simulink subsystem "Strecke"  (R2021b)
settings: Solver=VariableStepAuto  StartTime=0.0  StopTime=10.0  RelTol=1e-3
undefined symbols (not defined in the file or in its folder): SimParam
settings Model: Creator=tim  LastModifiedBy=tim

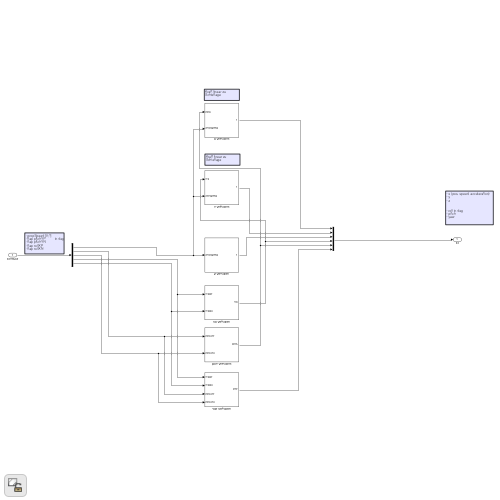
[thumbnail: Simulink's stored preview of the top-level diagram]
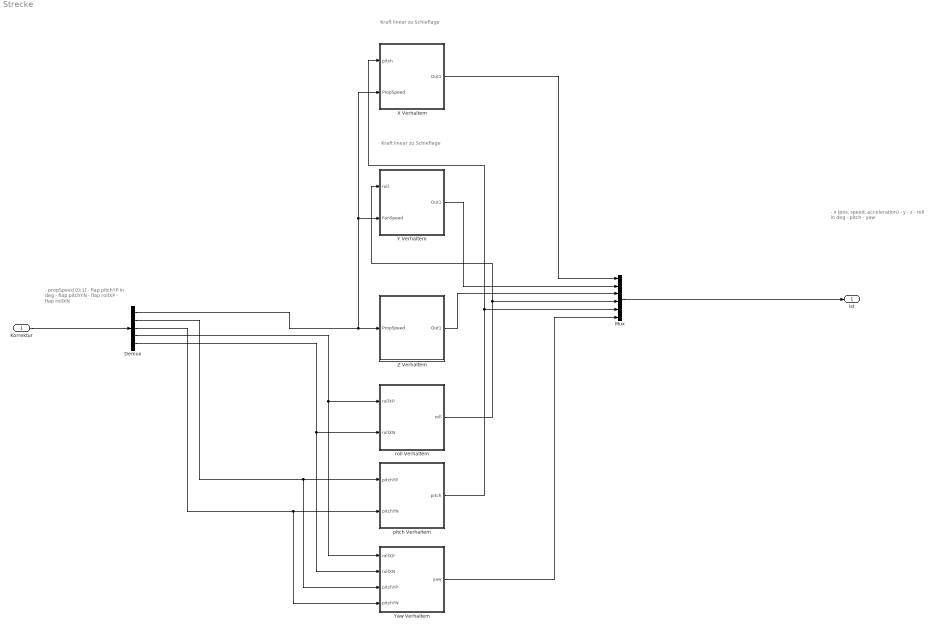
== system Strecke ==
  note: Kraft linear zu
      | Schieflage
  note: - propSpeed [0;1]
      | - flap pitchYP          in deg
      | - flap pitchYN
      | - flap rollXP
      | - flap rollXN
  note: - x (pos, speed, acceleration)
      | - y
      | - z
      |
      |
      | - roll in deg
      | - pitch
      | - yaw
  note: Kraft linear zu
      | Schieflage
  Korrektur : Inport
  Demux : Demux  Outputs=5
  Mux : Mux  Inputs=6
  X Verhaltem : Subsystem
  Y Verhaltem : Subsystem
  Yaw Verhaltem : Subsystem
  Z Verhaltem : Subsystem
  pitch Verhaltem : Subsystem
  roll Verhaltem : Subsystem
  ist : Outport
  wires:
  Demux/1 -> Z Verhaltem/1(PropSpeed), Y Verhaltem/2(FanSpeed), X Verhaltem/2(PropSpeed)
  Z Verhaltem/1(Out1) -> Mux/3
  Korrektur/1 -> Demux/1
  X Verhaltem/1(Out1) -> Mux/1
  Y Verhaltem/1(Out1) -> Mux/2
  Demux/2 -> pitch Verhaltem/1(pitchYP), Yaw Verhaltem/3(pitchYP)
  Demux/3 -> pitch Verhaltem/2(pitchYN), Yaw Verhaltem/4(pitchYN)
  Demux/4 -> roll Verhaltem/1(rollXP), Yaw Verhaltem/1(rollXP)
  Demux/5 -> roll Verhaltem/2(rollXN), Yaw Verhaltem/2(rollXN)
  roll Verhaltem/1(roll) -> Y Verhaltem/1(roll), Mux/4
  Yaw Verhaltem/1(yaw) -> Mux/6
  pitch Verhaltem/1(pitch) -> X Verhaltem/1(pitch), Mux/5
  Mux/1 -> ist/1

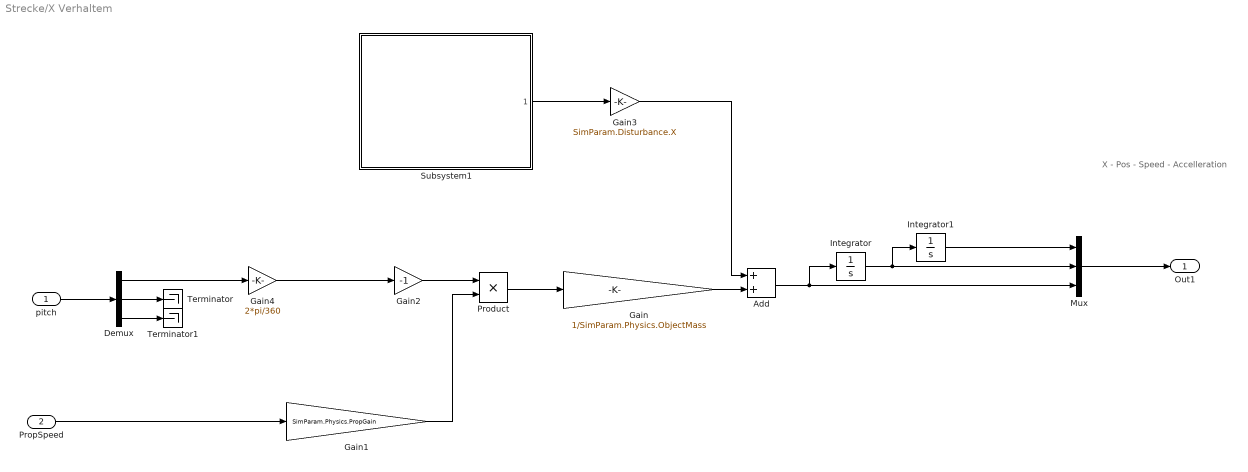
== system Strecke/X Verhaltem ==
  note: X
      | - Pos
      | - Speed
      | - Accelleration
  pitch : Inport
  PropSpeed : Inport  Port=2
  Add : Sum
  Demux : Demux  Outputs=3
  Gain : Gain  Gain=1/SimParam.Physics.ObjectMass
  Gain1 : Gain  Gain=SimParam.Physics.PropGain
  Gain2 : Gain  Gain=-1
  Gain3 : Gain  Gain=SimParam.Disturbance.X
  Gain4 : Gain  Gain=2*pi/360
  Integrator : Integrator
  Integrator1 : Integrator
  Mux : Mux  Inputs=3
  Product : Product
  Subsystem1 : Subsystem  ReferencedSubsystem=Disturbance
  Terminator : Terminator
  Terminator1 : Terminator
  Out1 : Outport
  wires:
  Gain2/1 -> Product/1
  Gain4/1 -> Gain2/1
  Gain1/1 -> Product/2
  PropSpeed/1 -> Gain1/1
  Gain3/1 -> Add/1
  Subsystem1/1 -> Gain3/1
  Gain/1 -> Add/2
  Demux/1 -> Gain4/1
  Demux/3 -> Terminator1/1
  Demux/2 -> Terminator/1
  Product/1 -> Gain/1
  Add/1 -> Mux/3, Integrator/1
  Integrator1/1 -> Mux/1
  Integrator/1 -> Mux/2, Integrator1/1
  pitch/1 -> Demux/1
  Mux/1 -> Out1/1

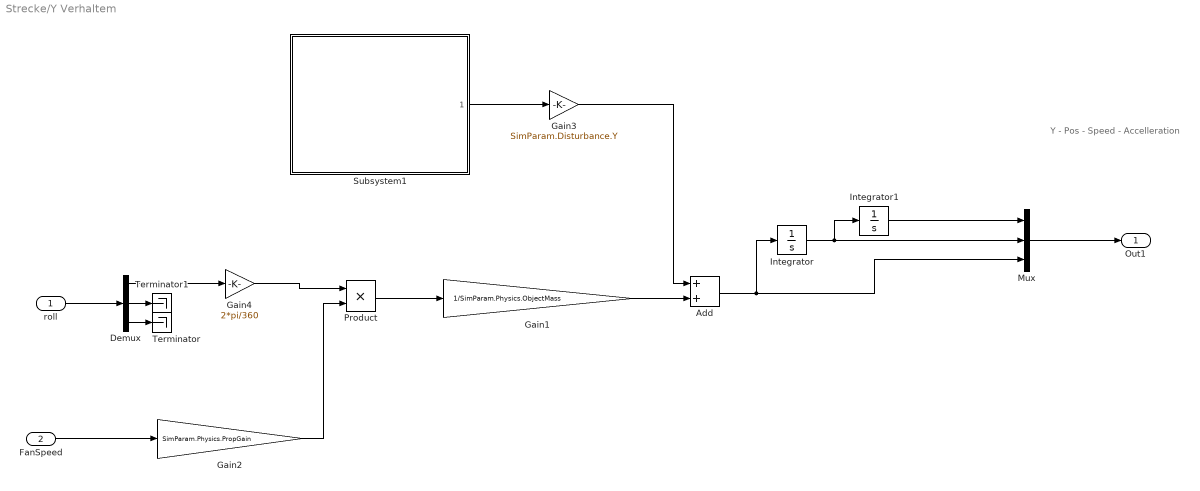
== system Strecke/Y Verhaltem ==
  note: Y
      | - Pos
      | - Speed
      | - Accelleration
  roll : Inport
  FanSpeed : Inport  Port=2
  Add : Sum
  Demux : Demux  Outputs=3
  Gain1 : Gain  Gain=1/SimParam.Physics.ObjectMass
  Gain2 : Gain  Gain=SimParam.Physics.PropGain
  Gain3 : Gain  Gain=SimParam.Disturbance.Y
  Gain4 : Gain  Gain=2*pi/360
  Integrator : Integrator
  Integrator1 : Integrator
  Mux : Mux  Inputs=3
  Product : Product
  Subsystem1 : Subsystem  ReferencedSubsystem=Disturbance
  Terminator : Terminator
  Terminator1 : Terminator
  Out1 : Outport
  wires:
  FanSpeed/1 -> Gain2/1
  Gain4/1 -> Product/1
  Gain2/1 -> Product/2
  Subsystem1/1 -> Gain3/1
  Gain3/1 -> Add/1
  Add/1 -> Mux/3, Integrator/1
  Demux/3 -> Terminator/1
  Demux/2 -> Terminator1/1
  Gain1/1 -> Add/2
  Product/1 -> Gain1/1
  Demux/1 -> Gain4/1
  Integrator1/1 -> Mux/1
  Integrator/1 -> Mux/2, Integrator1/1
  roll/1 -> Demux/1
  Mux/1 -> Out1/1

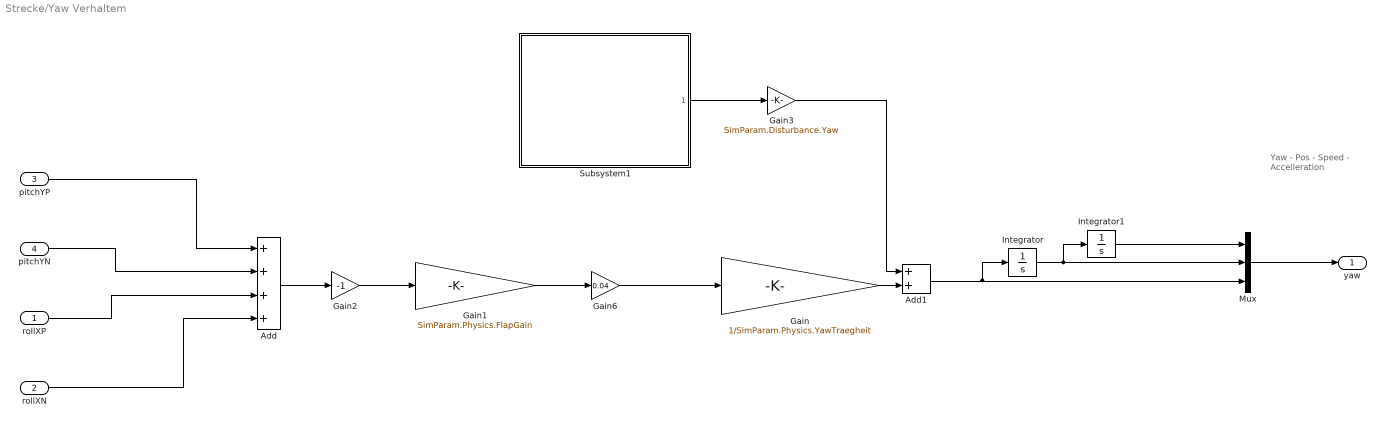
== system Strecke/Yaw Verhaltem ==
  note: Yaw
      | - Pos
      | - Speed
      | - Accelleration
  rollXP : Inport
  rollXN : Inport  Port=2
  pitchYP : Inport  Port=3
  pitchYN : Inport  Port=4
  Add : Sum  Inputs=++++
  Add1 : Sum
  Gain : Gain  Gain=1/SimParam.Physics.YawTraegheit
  Gain1 : Gain  Gain=SimParam.Physics.FlapGain
  Gain2 : Gain  Gain=-1
  Gain3 : Gain  Gain=SimParam.Disturbance.Yaw
  Gain6 : Gain  Gain=0.04
  Integrator : Integrator
  Integrator1 : Integrator
  Mux : Mux  Inputs=3
  Subsystem1 : Subsystem  ReferencedSubsystem=Disturbance
  yaw : Outport
  wires:
  Gain2/1 -> Gain1/1
  Gain/1 -> Add1/2
  Subsystem1/1 -> Gain3/1
  Gain3/1 -> Add1/1
  Gain6/1 -> Gain/1
  Add/1 -> Gain2/1
  Mux/1 -> yaw/1
  rollXN/1 -> Add/4
  rollXP/1 -> Add/3
  pitchYN/1 -> Add/2
  pitchYP/1 -> Add/1
  Add1/1 -> Integrator/1, Mux/3
  Gain1/1 -> Gain6/1
  Integrator1/1 -> Mux/1
  Integrator/1 -> Mux/2, Integrator1/1

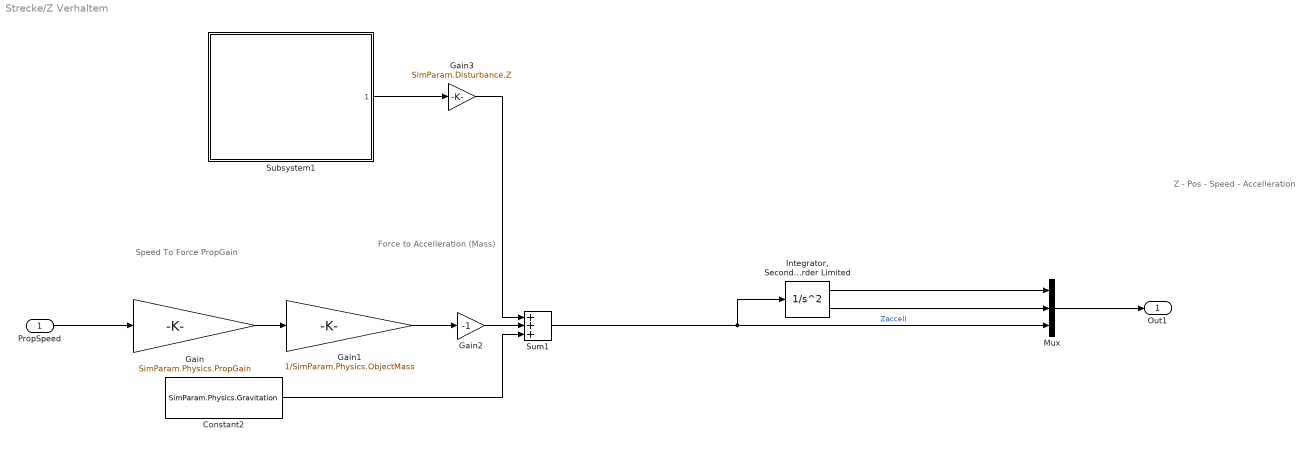
== system Strecke/Z Verhaltem ==
  note: Force to Accelleration
      | (Mass)
  note: Z
      | - Pos
      | - Speed
      | - Accelleration
  note: Speed To Force
      | PropGain
  PropSpeed : Inport
  Constant2 : Constant  Value=SimParam.Physics.Gravitation
  Gain : Gain  Gain=SimParam.Physics.PropGain
  Gain1 : Gain  Gain=1/SimParam.Physics.ObjectMass
  Gain2 : Gain  Gain=-1
  Gain3 : Gain  Gain=SimParam.Disturbance.Z
  "Integrator, Second-Order Limited" : SecondOrderIntegrator  LimitX=on  UpperLimitX=0  LowerLimitX=-1000000  LimitDXDT=on
  Mux : Mux  Inputs=3
  Subsystem1 : Subsystem  ReferencedSubsystem=Disturbance
  Sum1 : Sum  Inputs=+++
  Out1 : Outport
  wires:
  Gain2/1 -> Sum1/2
  Gain/1 -> Gain1/1
  Subsystem1/1 -> Gain3/1
  Gain3/1 -> Sum1/1
  PropSpeed/1 -> Gain/1
  Gain1/1 -> Gain2/1
  "Integrator, Second-Order Limited"/2 -> Mux/2
  "Integrator, Second-Order Limited"/1 -> Mux/1
  Sum1/1 -> "Integrator, Second-Order Limited"/1, Mux/3  "Zaccell"
  Constant2/1 -> Sum1/3
  Mux/1 -> Out1/1

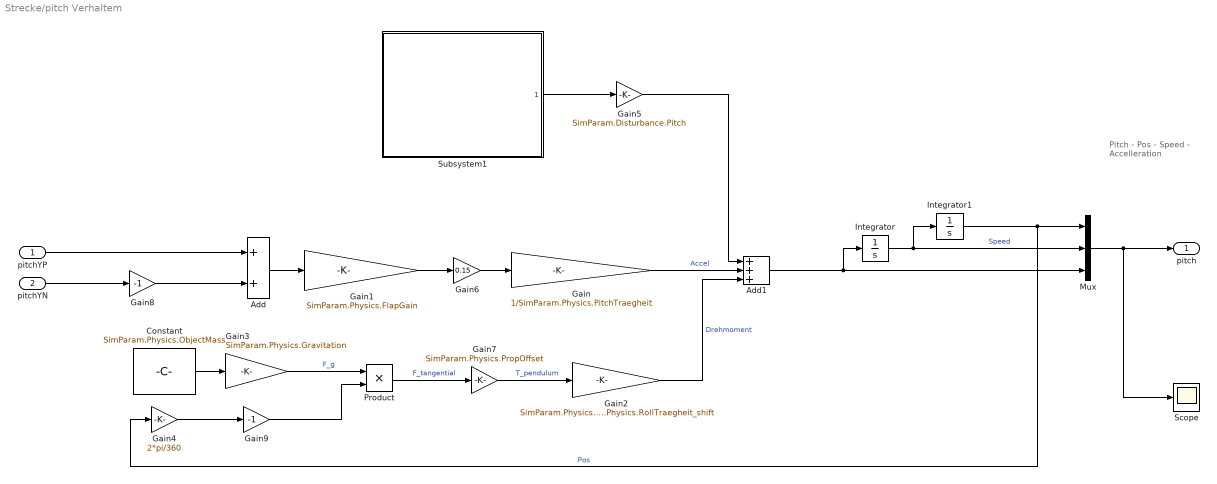
== system Strecke/pitch Verhaltem ==
  note: Pitch
      | - Pos
      | - Speed
      | - Accelleration
  pitchYP : Inport
  pitchYN : Inport  Port=2
  Add : Sum
  Add1 : Sum  Inputs=+++
  Constant : Constant  Value=SimParam.Physics.ObjectMass
  Gain : Gain  Gain=1/SimParam.Physics.PitchTraegheit
  Gain1 : Gain  Gain=SimParam.Physics.FlapGain
  Gain2 : Gain  Gain=SimParam.Physics.PropOffset/SimParam.Physics.RollTraegheit_shift
  Gain3 : Gain  Gain=SimParam.Physics.Gravitation
  Gain4 : Gain  Gain=2*pi/360
  Gain5 : Gain  Gain=SimParam.Disturbance.Pitch
  Gain6 : Gain  Gain=0.15
  Gain7 : Gain  Gain=SimParam.Physics.PropOffset
  Gain8 : Gain  Gain=-1
  Gain9 : Gain  Gain=-1
  Integrator : Integrator
  Integrator1 : Integrator
  Mux : Mux  Inputs=3
  Product : Product
  Scope : Scope
  Subsystem1 : Subsystem  ReferencedSubsystem=Disturbance
  pitch : Outport
  wires:
  Gain9/1 -> Product/2
  Gain8/1 -> Add/2
  Gain7/1 -> Gain2/1  "T_pendulum"
  Gain6/1 -> Gain/1
  Gain4/1 -> Gain9/1
  Subsystem1/1 -> Gain5/1
  Gain5/1 -> Add1/1
  Add/1 -> Gain1/1
  Product/1 -> Gain7/1  "F_tangential"
  Gain3/1 -> Product/1  "F_g"
  Constant/1 -> Gain3/1
  Gain2/1 -> Add1/3  "Drehmoment"
  Gain/1 -> Add1/2  "Accel"
  Add1/1 -> Mux/3, Integrator/1
  pitchYN/1 -> Gain8/1
  Gain1/1 -> Gain6/1
  Integrator1/1 -> Mux/1, Gain4/1  "Pos"
  Integrator/1 -> Mux/2, Integrator1/1  "Speed"
  pitchYP/1 -> Add/1
  Mux/1 -> Scope/1, pitch/1

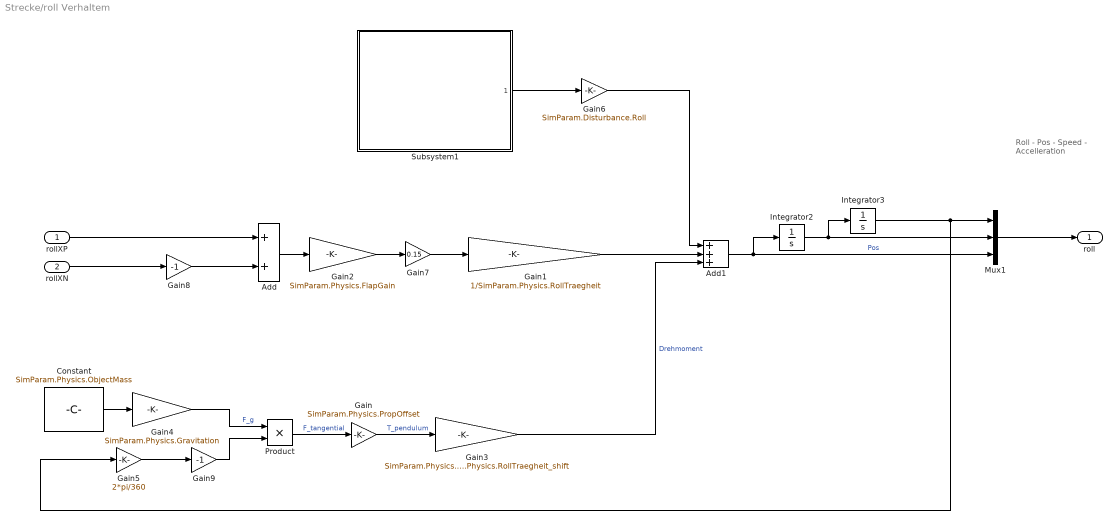
== system Strecke/roll Verhaltem ==
  note: Roll
      | - Pos
      | - Speed
      | - Accelleration
  rollXP : Inport
  rollXN : Inport  Port=2
  Add : Sum
  Add1 : Sum  Inputs=+++
  Constant : Constant  Value=SimParam.Physics.ObjectMass
  Gain : Gain  Gain=SimParam.Physics.PropOffset
  Gain1 : Gain  Gain=1/SimParam.Physics.RollTraegheit
  Gain2 : Gain  Gain=SimParam.Physics.FlapGain
  Gain3 : Gain  Gain=SimParam.Physics.PropOffset/SimParam.Physics.RollTraegheit_shift
  Gain4 : Gain  Gain=SimParam.Physics.Gravitation
  Gain5 : Gain  Gain=2*pi/360
  Gain6 : Gain  Gain=SimParam.Disturbance.Roll
  Gain7 : Gain  Gain=0.15
  Gain8 : Gain  Gain=-1
  Gain9 : Gain  Gain=-1
  Integrator2 : Integrator
  Integrator3 : Integrator
  Mux1 : Mux  Inputs=3
  Product : Product
  Subsystem1 : Subsystem  ReferencedSubsystem=Disturbance
  roll : Outport
  wires:
  Gain9/1 -> Product/2
  Gain8/1 -> Add/2
  Gain/1 -> Gain3/1  "T_pendulum"
  Gain7/1 -> Gain1/1
  Gain5/1 -> Gain9/1
  Subsystem1/1 -> Gain6/1
  Gain6/1 -> Add1/1
  Add/1 -> Gain2/1
  Integrator2/1 -> Mux1/2, Integrator3/1
  Gain1/1 -> Add1/2
  Gain4/1 -> Product/1  "F_g"
  Integrator3/1 -> Mux1/1, Gain5/1
  Add1/1 -> Integrator2/1, Mux1/3  "Pos"
  Gain3/1 -> Add1/3  "Drehmoment"
  Constant/1 -> Gain4/1
  Product/1 -> Gain/1  "F_tangential"
  rollXP/1 -> Add/1
  Gain2/1 -> Gain7/1
  Mux1/1 -> roll/1
  rollXN/1 -> Gain8/1
